simulink model "cascade_form"  (R2020a)
settings: Solver=VariableStepAuto  StartTime=0.0  StopTime=10.0  RelTol=1e-3
libraries: dspsrcs4 x1
settings Model: Creator=kolep  LastModifiedBy=kolep

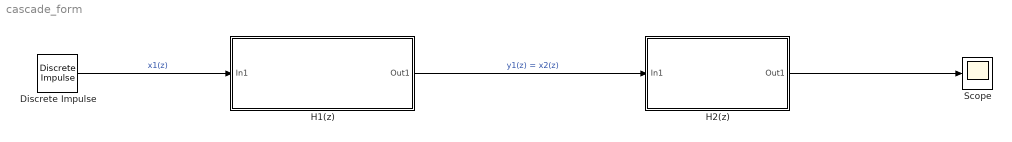
== system cascade_form ==
  Discrete Impulse : dspsrcs4/Discrete  Impulse  Delay=0  SampleTime=1  FrameSample=1  OutputFrames=off  dataType=double  isSigned=on  wordLen=16  udDataType=sfix(16)  fracBitsMode=Best precision  numFracBits=15  OutDataTypeStr=double  LastOutDataTypeStr=double
  H1(z) : Subsystem
  H2(z) : Subsystem
  Scope : Scope
  wires:
  Discrete Impulse/1 -> H1(z)/1(In1)  "x1(z)"
  H1(z)/1(Out1) -> H2(z)/1(In1)  "y1(z) = x2(z)"
  H2(z)/1(Out1) -> Scope/1

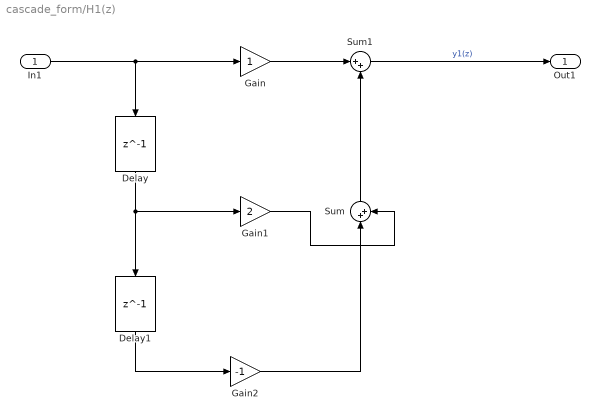
== system cascade_form/H1(z) ==
  In1 : Inport
  Delay : Delay  DelayLength=1  InputProcessing=Columns as channels (frame based)
  Delay1 : Delay  DelayLength=1  InputProcessing=Columns as channels (frame based)
  Gain : Gain
  Gain1 : Gain  Gain=2
  Gain2 : Gain  Gain=-1
  Sum : Sum  Inputs=|++
  Sum1 : Sum  Inputs=|++
  Out1 : Outport
  wires:
  Gain/1 -> Sum1/1
  In1/1 -> Delay/1, Gain/1
  Gain2/1 -> Sum/1
  Gain1/1 -> Sum/2
  Delay/1 -> Delay1/1, Gain1/1
  Delay1/1 -> Gain2/1
  Sum/1 -> Sum1/2
  Sum1/1 -> Out1/1  "y1(z)"

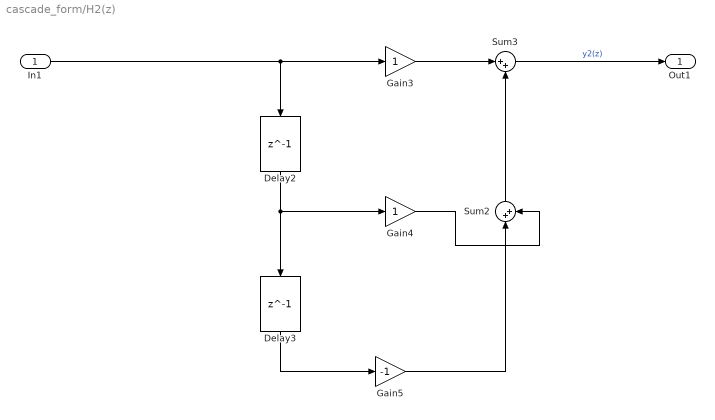
== system cascade_form/H2(z) ==
  In1 : Inport
  Delay2 : Delay  DelayLength=1  InputProcessing=Columns as channels (frame based)
  Delay3 : Delay  DelayLength=1  InputProcessing=Columns as channels (frame based)
  Gain3 : Gain
  Gain4 : Gain
  Gain5 : Gain  Gain=-1
  Sum2 : Sum  Inputs=|++
  Sum3 : Sum  Inputs=|++
  Out1 : Outport
  wires:
  Delay3/1 -> Gain5/1
  Gain3/1 -> Sum3/1
  Gain4/1 -> Sum2/2
  In1/1 -> Delay2/1, Gain3/1
  Sum3/1 -> Out1/1  "y2(z)"
  Sum2/1 -> Sum3/2
  Delay2/1 -> Delay3/1, Gain4/1
  Gain5/1 -> Sum2/1
